simulink model "adc_sst_v7"  (R2012b)
settings: Solver=FixedStepDiscrete  SolverMode=SingleTasking  StartTime=0.0  StopTime=10000  FixedStep=1  RelTol=1e-3
libraries: xbsIndex_r4 x1894, casper_library_misc x43, dspsigops x32, xps_library x6
(part 3 of 19)

== system adc_sst_v7/adc1 ==
  Pulse Generator : DiscretePulseGenerator  Period=1000000000  PhaseDelay=10
  Sine Wave : Sin  SineType=Sample based  Amplitude=0.8  Bias=0.01  Samples=32  SampleTime=1
  asiaa_adc5g : Subsystem  Tag=xps:adc5g  AncestorBlock=xps_library/ADCs/asiaa_adc5g  mask(adc5g){input_mode=One-channel -- A, adc_brd=ZDOK 1, demux=1:1, adc_bit_width=8, adc_clk_rate=Fe/2, using_ctrl=on, test_ramp=off}
      mask prompts: input_mode "Input mode:"; adc_brd "ADC Board"; demux "Internal demux"; adc_bit_width "ADC Resolution (bits):"; adc_clk_rate "ADC Clock Rate (MHz):"; using_ctrl "use control"; test_ramp "start in test ramp mode"
      mask help:
      | Interface for the ASIAA 5 GSps ADC. Supports interleaving all four
      | cores using either input A or C, or interleaving two-cores each for
      | A and C. The hardware itself comes in two versions:
      |
      | DMUX 1:2 -- 4-bit samples, 4 parallel streams
      | DMUX 1:1 -- 8-bit samples, 2 parallel streams
      |
      | In either configuration this block will output 8 parallel streams
      | but the underlying interface, and the bitwidth of the samples,
      | will be different.
      mask init: same as adc_sst_v7/adc0/asiaa_adc5g
      mask TypeOptions input_mode: One-channel -- A | One-channel -- C | Two-channel -- A&C
      mask TypeOptions adc_brd: ZDOK 0 | ZDOK 1
      mask TypeOptions demux: 1:1 | 1:2
      mask Callback demux:
      | demux = get_param(gcb,'demux');
      | if(strcmp(demux,'1:1')),
      |     set_param(gcb, 'adc_bit_width', '8')
      | elseif(strcmp(demux, '1:2')),
      |     set_param(gcb, 'adc_bit_width', '4');
      | else
      | end
  bus_create : Subsystem  AncestorBlock=casper_library_flow_control/bus_create  mask(bus_create){inputNum=16}
      mask prompts: inputNum "Number of inputs:"
      mask init:
      | bus_create_init(gcb,...
      |     'inputNum', inputNum);
  converter : Subsystem
  converter1 : Subsystem
  converter10 : Subsystem
  converter11 : Subsystem
  converter12 : Subsystem
  converter13 : Subsystem
  converter14 : Subsystem
  converter16 : Subsystem
  converter2 : Subsystem
  converter3 : Subsystem
  converter4 : Subsystem
  converter5 : Subsystem
  converter6 : Subsystem
  converter7 : Subsystem
  converter8 : Subsystem
  converter9 : Subsystem
  pipeline1 : Subsystem  AncestorBlock=casper_library_delays/pipeline  mask(pipeline){latency=2}
      mask help:
      | An explicitly laid-out delay line to avoid mapping to SRL16s
      | for use in pipelining to help achieve timing closure.
      mask init:
      | pipeline_init(gcb,'latency',latency);
      settings: AttributesFormatString=Latency = %<latency>
      mask Display:
      | port_label('input', 1, 'd');
      | port_label('output', 1, 'q');
      | disp(['Z^-', num2str(latency)]);
  pipeline61 : Subsystem  AncestorBlock=casper_library_delays/pipeline  mask(pipeline){latency=2}
      mask help:
      | An explicitly laid-out delay line to avoid mapping to SRL16s
      | for use in pipelining to help achieve timing closure.
      mask init:
      | pipeline_init(gcb,'latency',latency);
      settings: AttributesFormatString=Latency = %<latency>
      mask Display:
      | port_label('input', 1, 'd');
      | port_label('output', 1, 'q');
      | disp(['Z^-', num2str(latency)]);
  dout : Outport
  sync_out : Outport  Port=2
  wires:
  asiaa_adc5g/5(a4) -> converter8/1(u8_0)
  asiaa_adc5g/6(a5) -> converter4/1(u8_0)
  asiaa_adc5g/16(a15) -> converter14/1(u8_0)
  asiaa_adc5g/12(a11) -> converter11/1(u8_0)
  asiaa_adc5g/4(a3) -> converter3/1(u8_0)
  asiaa_adc5g/2(a1) -> converter1/1(u8_0)
  asiaa_adc5g/15(a14) -> converter13/1(u8_0)
  Pulse Generator/1 -> asiaa_adc5g/2(sim_sync)
  asiaa_adc5g/14(a13) -> converter16/1(u8_0)
  asiaa_adc5g/7(a6) -> converter5/1(u8_0)
  asiaa_adc5g/13(a12) -> converter12/1(u8_0)
  asiaa_adc5g/10(a9) -> converter9/1(u8_0)
  asiaa_adc5g/1(a0) -> converter/1(u8_0)
  asiaa_adc5g/11(a10) -> converter10/1(u8_0)
  asiaa_adc5g/3(a2) -> converter2/1(u8_0)
  asiaa_adc5g/8(a7) -> converter6/1(u8_0)
  asiaa_adc5g/9(a8) -> converter7/1(u8_0)
  Sine Wave/1 -> asiaa_adc5g/1(sim_a)
  converter/1(s8_7) -> bus_create/1(in1)
  asiaa_adc5g/17(sync_out) -> pipeline1/1(d)
  converter14/1(s8_7) -> bus_create/16(in16)
  converter1/1(s8_7) -> bus_create/2(in2)
  converter2/1(s8_7) -> bus_create/3(in3)
  converter3/1(s8_7) -> bus_create/4(in4)
  converter8/1(s8_7) -> bus_create/5(in5)
  converter4/1(s8_7) -> bus_create/6(in6)
  converter5/1(s8_7) -> bus_create/7(in7)
  converter6/1(s8_7) -> bus_create/8(in8)
  converter7/1(s8_7) -> bus_create/9(in9)
  converter9/1(s8_7) -> bus_create/10(in10)
  converter10/1(s8_7) -> bus_create/11(in11)
  converter11/1(s8_7) -> bus_create/12(in12)
  converter12/1(s8_7) -> bus_create/13(in13)
  converter16/1(s8_7) -> bus_create/14(in14)
  converter13/1(s8_7) -> bus_create/15(in15)
  bus_create/1(bus_out) -> pipeline61/1(d)
  pipeline61/1(q) -> dout/1
  pipeline1/1(q) -> sync_out/1

== system adc_sst_v7/armed_pps ==
  pps_in : Inport
  arm : Inport  Port=2
  edge_detect1 : Subsystem  AncestorBlock=casper_library_misc/edge_detect  mask(edge_detect){edge=Rising, polarity=Active High, x_in=[0 0.08 0.08 0.16 0.16 0.24 0.24 0.32 0.32 0.4], y_in=[-1 -1  1  1  1  1  1  1  1  1], x_out=[0.6 0.68 0.68 0.76 0.76 0.84 0.84 0.92 0.92 1], y_out=[-1 -1  1  1 -1 -1 -1 -1 -1 -1]}
      mask prompts: edge "Edge Type"; polarity "Output Polarity"; x_in "Input X Positions"; y_in "Input Y Positions"; x_out "Output X Positions"; y_out "Output Y Positions"
      mask help: Output is active for one-cycle after each edge of the specified type (i.e. rising, falling or both).
      mask init: same as adc_sst_v7/edge_detect2
      settings: AttributesFormatString=|
      | rising edges
      | active high
      mask Help: Output is active for one-cycle after each edge of the specified type (i.e. rising, falling, or both).  Latency is zero.
      mask TypeOptions edge: Rising | Falling | Both
      mask TypeOptions polarity: Active High | Active Low
      mask Display:
      | plot(x_in_num,0.5+y_in_num*0.2);
      | plot(x_out_num,0.5+y_out_num*0.2);
  log_arm_delay1 : xbsIndex_r4/Delay  rst=off  infoeditControl=Selection of Reset will increase slice count due to use of real FFs and instead of SRLs  en=off  latency=1  dbl_ovrd=off  reg_retiming=on  block_type=delay
      settings: xl_area=[0, 0, 0, 0, 0, 0, 0]
  log_arm_delay2 : xbsIndex_r4/Delay  rst=off  infoeditControl=Selection of Reset will increase slice count due to use of real FFs and instead of SRLs  en=off  latency=1  dbl_ovrd=off  reg_retiming=on  block_type=delay
      settings: xl_area=[0, 0, 0, 0, 0, 0, 0]
  log_arm_pps : xbsIndex_r4/Logical  logical_function=AND  inputs=2  en=off  latency=1  precision=Full  arith_type=Unsigned  n_bits=8  bin_pt=2  align_bp=on  dbl_ovrd=off  block_type=logical
      settings: xl_area=[0, 0, 0, 0, 0, 0, 0]
  pipeline60 : Subsystem  AncestorBlock=casper_library_delays/pipeline  mask(pipeline){latency=2}
      mask help:
      | An explicitly laid-out delay line to avoid mapping to SRL16s
      | for use in pipelining to help achieve timing closure.
      mask init:
      | pipeline_init(gcb,'latency',latency);
      settings: AttributesFormatString=Latency = %<latency>
      mask Display:
      | port_label('input', 1, 'd');
      | port_label('output', 1, 'q');
      | disp(['Z^-', num2str(latency)]);
  reg_reset_arm : xbsIndex_r4/Register  init=0  rst=on  en=on  dbl_ovrd=off  block_type=register
      settings: xl_area=[0, 0, 0, 0, 0, 0, 0]
  reg_reset_const : xbsIndex_r4/Constant  const=1  gui_display_data_type=Fixed-point  arith_type=Boolean  n_bits=16  bin_pt=14  preci_type=Single  exp_width=8  frac_width=24  explicit_period=off  period=1  equ=P=C  opselect=C  inp2=PCIN>>17  opr=+  inp1=P  carry=CIN  dbl_ovrd=off  block_type=constant
      settings: block_version=11.4
  pps_out : Outport
  wires:
  reg_reset_arm/1 -> log_arm_delay2/1
  pps_in/1 -> log_arm_delay1/1
  log_arm_pps/1 -> pipeline60/1(d), reg_reset_arm/2
  arm/1 -> edge_detect1/1(in)
  edge_detect1/1(out) -> reg_reset_arm/3
  reg_reset_const/1 -> reg_reset_arm/1
  log_arm_delay1/1 -> log_arm_pps/1
  log_arm_delay2/1 -> log_arm_pps/2
  pipeline60/1(q) -> pps_out/1

== system adc_sst_v7/armed_sync_cnt ==
  out_reg : Inport
  adc_sst_v7_armed_sync_cnt_user_data_in : xbsIndex_r4/Gateway Out  inherit_from_input=off  hdl_port=on  timing_constraint=None  locs_specified=off  LOCs={}  UseAsDAC=off  DACChannel='1'  block_type=gatewayout
  assert_reg : xbsIndex_r4/Assert  assert_type=on  type_source=Explicitly  gui_display_data_type=Fixed-point  arith_type=Unsigned  n_bits=32  bin_pt=0  preci_type=Single  exp_width=8  frac_width=24  assert_rate=off  rate_source=Explicitly  period=1  output_port=on  block_type=assert
  cast_gw : xbsIndex_r4/Convert  gui_display_data_type=Fixed-point  arith_type=Unsigned  n_bits=32  bin_pt=0  float_type=Single  exp_bits=8  fraction_bits=24  quantization=Truncate  overflow=Wrap  en=off  latency=0  dbl_ovrd=off  pipeline=off  block_type=convert
  io_delay : xbsIndex_r4/Delay  rst=off  infoeditControl=Selection of Reset will increase slice count due to use of real FFs and instead of SRLs  en=off  latency=0  dbl_ovrd=off  reg_retiming=on  block_type=delay
  reint1 : xbsIndex_r4/Reinterpret  force_arith_type=on  arith_type=Unsigned  force_bin_pt=on  bin_pt=0  block_type=reinterpret
  sim_out : Outport
  wires:
  io_delay/1 -> cast_gw/1
  cast_gw/1 -> adc_sst_v7_armed_sync_cnt_user_data_in/1
  adc_sst_v7_armed_sync_cnt_user_data_in/1 -> sim_out/1
  out_reg/1 -> assert_reg/1
  assert_reg/1 -> reint1/1
  reint1/1 -> io_delay/1

== system adc_sst_v7/cnt_rst ==
  sim_1 : Inport
  adc_sst_v7_cnt_rst_user_data_out : xbsIndex_r4/Gateway In  gui_display_data_type=Fixed-point  arith_type=Unsigned  n_bits=32  bin_pt=0  preci_type=Single  exp_width=8  frac_width=24  quantization="Round  (unbiased: +/- Inf)"  overflow=Saturate  period=1  dbl_ovrd=off  timing_constraint=None  locs_specified=off  LOCs={}  UseAsADC=off  ADCChannel='1'  inherit_from_input=off  hdl_port=on  block_type=gatewayin
  io_delay : xbsIndex_r4/Delay  rst=off  infoeditControl=Selection of Reset will increase slice count due to use of real FFs and instead of SRLs  en=off  latency=0  dbl_ovrd=off  reg_retiming=on  block_type=delay
  reint1 : xbsIndex_r4/Reinterpret  force_arith_type=on  arith_type=Unsigned  force_bin_pt=on  bin_pt=0  block_type=reinterpret
  slice_reg : xbsIndex_r4/Slice  nbits=32  boolean_output=off  mode=Lower Bit Location + Width  bit1=0  base1=MSB of Input  bit0=0  base0=LSB of Input  dbl_ovrd=off  block_type=slice
  in_reg : Outport
  wires:
  adc_sst_v7_cnt_rst_user_data_out/1 -> io_delay/1
  sim_1/1 -> adc_sst_v7_cnt_rst_user_data_out/1
  io_delay/1 -> slice_reg/1
  slice_reg/1 -> reint1/1
  reint1/1 -> in_reg/1

== system adc_sst_v7/edge_detect2 ==
  in : Inport
  Delay : xbsIndex_r4/Delay  rst=off  infoeditControl=Selection of Reset will increase slice count due to use of real FFs and instead of SRLs  en=off  latency=1  dbl_ovrd=off  reg_retiming=off  block_type=delay
      settings: xl_area=[0, 0, 0, 0, 0, 0, 0]
  Inverter : xbsIndex_r4/Inverter  en=off  latency=0  dbl_ovrd=off  block_type=inv
      settings: xl_area=[0, 0, 0, 0, 0, 0, 0]
  edge_op : xbsIndex_r4/Logical  logical_function=NOR  inputs=2  en=off  latency=0  precision=Full  arith_type=Unsigned  n_bits=8  bin_pt=2  align_bp=on  dbl_ovrd=off  block_type=logical
      settings: xl_area=[0, 0, 0, 0, 0, 0, 0]
  out : Outport
  wires:
  Inverter/1 -> edge_op/1
  edge_op/1 -> out/1
  in/1 -> Inverter/1, Delay/1
  Delay/1 -> edge_op/2
